simulink model "pre_Q"  (R2019b)
settings: Solver=VariableStepAuto  StartTime=0.0  StopTime=200  RelTol=1e-3
libraries: cstblocks x1
settings Model: Creator=amirhosein  LastModifiedBy=amirhosein

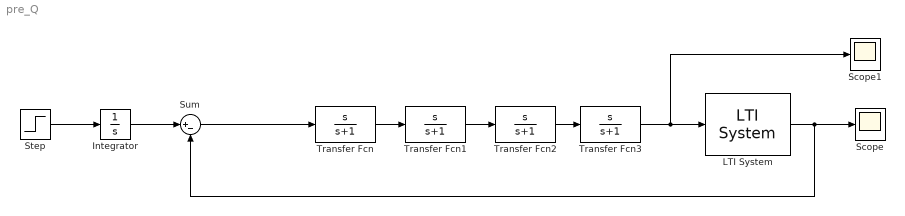
== system pre_Q ==
  Integrator : Integrator
  LTI System : cstblocks/LTI System  sys=Gp  IC=[]
  Scope : Scope
  Scope1 : Scope
  Step : Step  Time=0  After=0.5  SampleTime=0.001
  Sum : Sum  Inputs=|+-
  Transfer Fcn{,1..3} (4 alike) : TransferFcn  Numerator=[1 0]  Denominator=[1 1]
  wires:
  Step/1 -> Integrator/1
  Integrator/1 -> Sum/1
  Sum/1 -> Transfer Fcn/1
  Transfer Fcn3/1 -> Scope1/1, LTI System/1
  Transfer Fcn2/1 -> Transfer Fcn3/1
  Transfer Fcn1/1 -> Transfer Fcn2/1
  LTI System/1 -> Scope/1, Sum/2
  Transfer Fcn/1 -> Transfer Fcn1/1
